simulink model "mainmodel"  (R2020a)
settings: Solver=VariableStepAuto  StartTime=0.0  StopTime=10.0  RelTol=1e-3
undefined symbols (not defined in the file): b, m
settings Model: Creator=Bhanu  LastModifiedBy=Bhanu

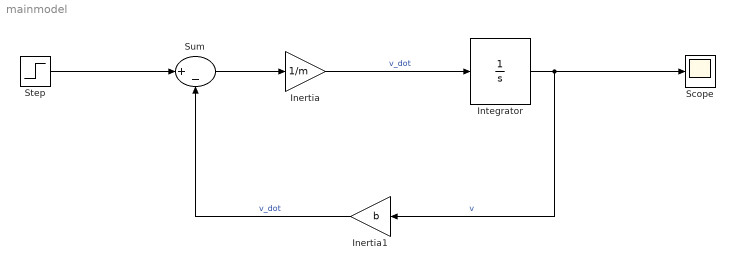
== system mainmodel ==
  Inertia : Gain  Gain=1/m
  Inertia1 : Gain  Gain=b
  Integrator : Integrator
  Scope : Scope
  Step : Step  Time=0  After=500  SampleTime=0
  Sum : Sum  Inputs=|+-
  wires:
  Inertia/1 -> Integrator/1  "v_dot"
  Integrator/1 -> Inertia1/1, Scope/1  "v"
  Sum/1 -> Inertia/1
  Inertia1/1 -> Sum/2  "v_dot"
  Step/1 -> Sum/1
